simulink model "order2_math_model"  (R2021a)
settings: Solver=FixedStepAuto  StartTime=0.0  StopTime=15  FixedStep=1e-3  RelTol=1e-3
values from neighbouring files (symbols this model uses):
  K = [23.4125   -0.5709   44.4357   22.3907 -283.0923  379.2252]    [order2_all_observer_sfun.m]    (also in order2_calc.m = K2)
  K_lqr = lqr(A,B,Q,R)    [order2_calc.m]
settings Model: Creator=cc  LastModifiedBy=cc

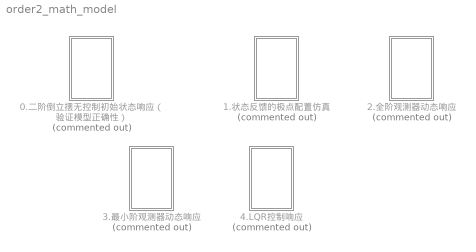
== system order2_math_model ==
  0.二阶倒立摆无控制初始状态响应（验证模型正确性） : Subsystem  Commented=on
  1.状态反馈的极点配置仿真 : Subsystem  Commented=on
  2.全阶观测器动态响应 : Subsystem  Commented=on
  3.最小阶观测器动态响应 : Subsystem  Commented=on
  4.LQR控制响应 : Subsystem  Commented=on

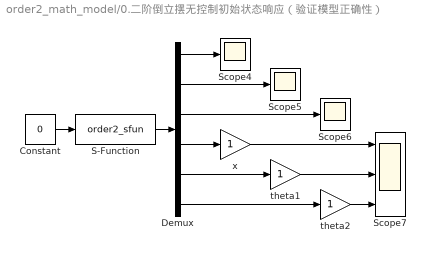
== system order2_math_model/0.二阶倒立摆无控制初始状态响应（验证模型正确性） ==
  Constant : Constant  Value=0
  Demux : Demux  Outputs=6
  S-Function : S-Function  FunctionName=order2_sfun  Parameters=0; 0; 0; 0; pi; 5/6*pi  SFunctionDeploymentMode=off  EnableBusSupport=off
  Scope4 : Scope
  Scope5 : Scope
  Scope6 : Scope
  Scope7 : Scope  NumInputPorts=3
  theta1 : Gain
  theta2 : Gain
  x : Gain
  wires:
  x/1 -> Scope7/1
  Demux/2 -> Scope5/1
  Constant/1 -> S-Function/1
  theta2/1 -> Scope7/3
  Demux/5 -> theta1/1
  theta1/1 -> Scope7/2
  Demux/6 -> theta2/1
  Demux/3 -> Scope6/1
  Demux/4 -> x/1
  S-Function/1 -> Demux/1
  Demux/1 -> Scope4/1

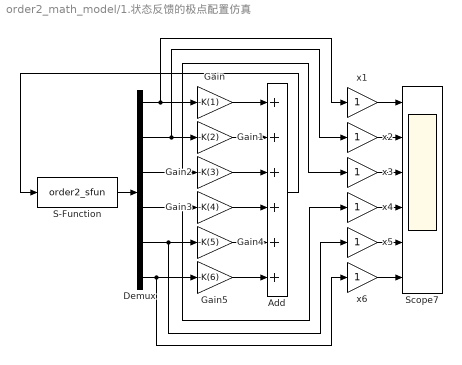
== system order2_math_model/1.状态反馈的极点配置仿真 ==
  Add : Sum  Inputs=++++++
  Demux : Demux  Outputs=6
  Gain : Gain  Gain=-K(1)
  Gain1 : Gain  Gain=-K(2)
  Gain2 : Gain  Gain=-K(3)
  Gain3 : Gain  Gain=-K(4)
  Gain4 : Gain  Gain=-K(5)
  Gain5 : Gain  Gain=-K(6)
  S-Function : S-Function  FunctionName=order2_sfun  Parameters=0; 0; 0; 0; 0; 5/180*pi  SFunctionDeploymentMode=off  EnableBusSupport=off
  Scope7 : Scope  NumInputPorts=6
  x{1..6} (6 alike) : Gain
  wires:
  S-Function/1 -> Demux/1
  Demux/1 -> x1/1, Gain/1
  Demux/2 -> Gain1/1, x2/1
  Demux/3 -> x3/1, Gain2/1
  Demux/4 -> x4/1, Gain3/1
  Demux/5 -> x5/1, Gain4/1
  Demux/6 -> x6/1, Gain5/1
  Gain/1 -> Add/1
  Gain1/1 -> Add/2
  Gain2/1 -> Add/3
  Gain3/1 -> Add/4
  Gain4/1 -> Add/5
  Gain5/1 -> Add/6
  Add/1 -> S-Function/1
  x1/1 -> Scope7/1
  x2/1 -> Scope7/2
  x3/1 -> Scope7/3
  x4/1 -> Scope7/4
  x5/1 -> Scope7/5
  x6/1 -> Scope7/6

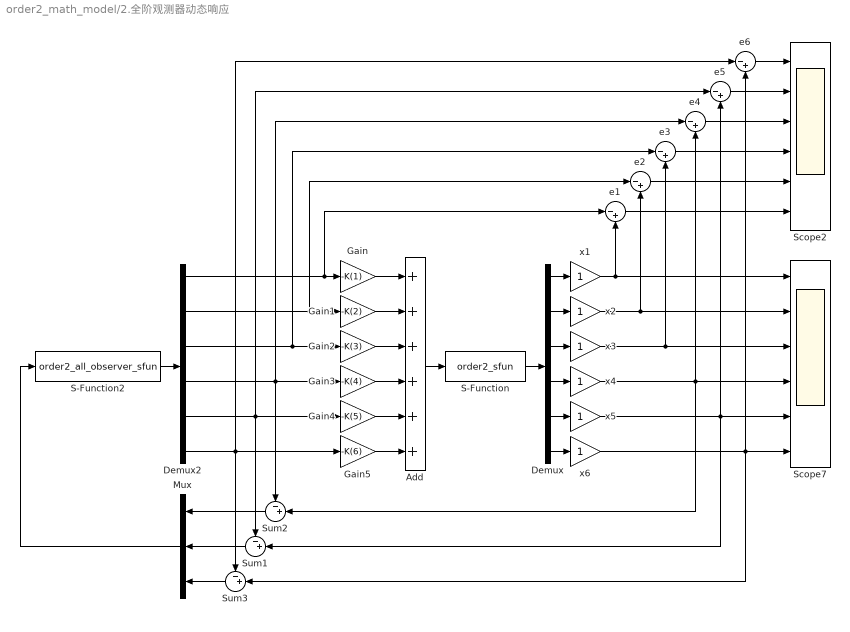
== system order2_math_model/2.全阶观测器动态响应 ==
  Add : Sum  Inputs=++++++
  Demux : Demux  Outputs=6
  Demux2 : Demux  Outputs=6
  Gain : Gain  Gain=-K(1)
  Gain1 : Gain  Gain=-K(2)
  Gain2 : Gain  Gain=-K(3)
  Gain3 : Gain  Gain=-K(4)
  Gain4 : Gain  Gain=-K(5)
  Gain5 : Gain  Gain=-K(6)
  Mux : Mux  Inputs=3
  S-Function : S-Function  FunctionName=order2_sfun  Parameters=0; 0; 0; 0; 0; 5/180*pi  SFunctionDeploymentMode=off  EnableBusSupport=off
  S-Function2 : S-Function  FunctionName=order2_all_observer_sfun  Parameters=0; 0; 0  SFunctionDeploymentMode=off  EnableBusSupport=off
  Scope2 : Scope  NumInputPorts=6
  Scope7 : Scope  NumInputPorts=6
  Sum1 : Sum  Inputs=-+|
  Sum2 : Sum  Inputs=-+|
  Sum3 : Sum  Inputs=-+|
  e{1..6} (6 alike) : Sum  Inputs=|-+
  x{1..6} (6 alike) : Gain
  wires:
  Demux/6 -> x6/1
  Gain/1 -> Add/1
  Gain1/1 -> Add/2
  Gain2/1 -> Add/3
  Gain3/1 -> Add/4
  Gain4/1 -> Add/5
  Gain5/1 -> Add/6
  Demux2/2 -> e2/1, Gain1/1
  Demux2/3 -> e3/1, Gain2/1
  Demux2/4 -> Gain3/1, e4/1, Sum2/1
  Demux2/5 -> Gain4/1, e5/1, Sum1/1
  Demux2/6 -> e6/1, Gain5/1, Sum3/1
  S-Function2/1 -> Demux2/1
  Demux2/1 -> e1/1, Gain/1
  Demux/4 -> x4/1
  Demux/5 -> x5/1
  Mux/1 -> S-Function2/1
  Demux/1 -> x1/1
  Demux/2 -> x2/1
  Demux/3 -> x3/1
  Sum2/1 -> Mux/1
  Sum1/1 -> Mux/2
  Sum3/1 -> Mux/3
  e3/1 -> Scope2/4
  e4/1 -> Scope2/3
  e5/1 -> Scope2/2
  e1/1 -> Scope2/6
  e2/1 -> Scope2/5
  e6/1 -> Scope2/1
  x1/1 -> Scope7/1, e1/2
  x3/1 -> Scope7/3, e3/2
  x4/1 -> Scope7/4, Sum2/2, e4/2
  x5/1 -> Scope7/5, Sum1/2, e5/2
  x6/1 -> Scope7/6, Sum3/2, e6/2
  x2/1 -> Scope7/2, e2/2
  Add/1 -> S-Function/1
  S-Function/1 -> Demux/1

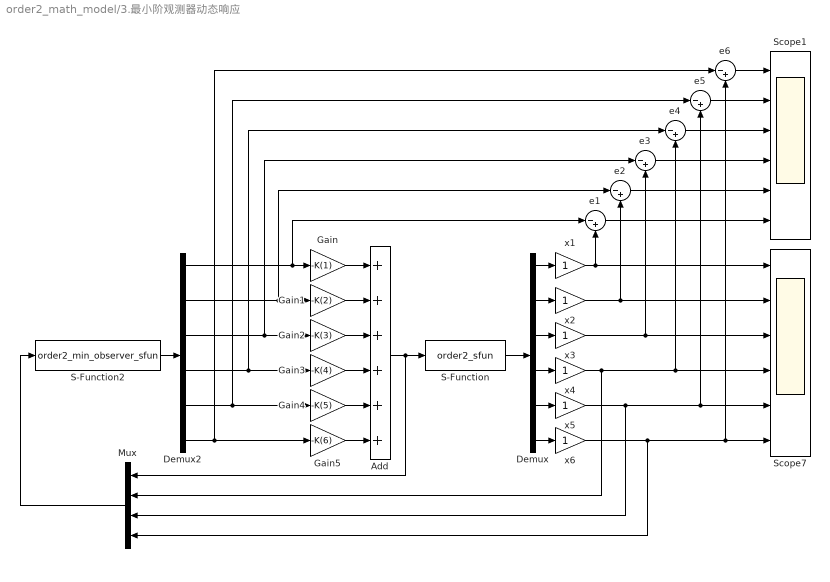
== system order2_math_model/3.最小阶观测器动态响应 ==
  Add : Sum  Inputs=++++++
  Demux : Demux  Outputs=6
  Demux2 : Demux  Outputs=6
  Gain : Gain  Gain=-K(1)
  Gain1 : Gain  Gain=-K(2)
  Gain2 : Gain  Gain=-K(3)
  Gain3 : Gain  Gain=-K(4)
  Gain4 : Gain  Gain=-K(5)
  Gain5 : Gain  Gain=-K(6)
  Mux : Mux
  S-Function : S-Function  FunctionName=order2_sfun  Parameters=0.05; 10/180*pi; 10/180*pi; 0; 0; 5/180*pi  SFunctionDeploymentMode=off  EnableBusSupport=off
  S-Function2 : S-Function  FunctionName=order2_min_observer_sfun  Parameters=0; 0; 5/180*pi; 0; 0; 0  SFunctionDeploymentMode=off  EnableBusSupport=off
  Scope1 : Scope  NumInputPorts=6
  Scope7 : Scope  NumInputPorts=6
  e{1..6} (6 alike) : Sum  Inputs=|-+
  x{1..6} (6 alike) : Gain
  wires:
  S-Function/1 -> Demux/1
  Demux/6 -> x6/1
  Gain/1 -> Add/1
  Gain1/1 -> Add/2
  Gain2/1 -> Add/3
  Gain3/1 -> Add/4
  Gain4/1 -> Add/5
  Gain5/1 -> Add/6
  Demux2/2 -> e2/1, Gain1/1
  Demux2/3 -> e3/1, Gain2/1
  Demux2/4 -> e4/1, Gain3/1
  Demux2/5 -> e5/1, Gain4/1
  Demux2/6 -> e6/1, Gain5/1
  S-Function2/1 -> Demux2/1
  Demux2/1 -> e1/1, Gain/1
  Demux/4 -> x4/1
  Demux/5 -> x5/1
  Add/1 -> S-Function/1, Mux/1
  Mux/1 -> S-Function2/1
  Demux/1 -> x1/1
  Demux/2 -> x2/1
  Demux/3 -> x3/1
  e1/1 -> Scope1/6
  e2/1 -> Scope1/5
  e3/1 -> Scope1/4
  e4/1 -> Scope1/3
  e5/1 -> Scope1/2
  x1/1 -> e1/2, Scope7/1
  x2/1 -> e2/2, Scope7/2
  x3/1 -> e3/2, Scope7/3
  x4/1 -> e4/2, Scope7/4, Mux/2
  x5/1 -> e5/2, Scope7/5, Mux/3
  x6/1 -> e6/2, Scope7/6, Mux/4
  e6/1 -> Scope1/1

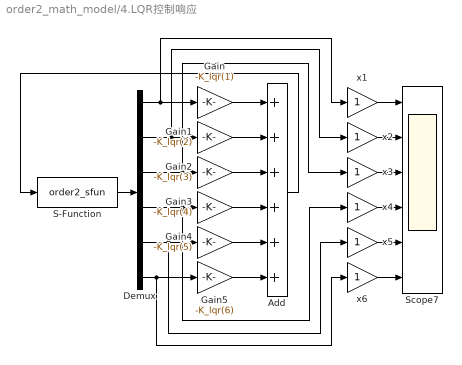
== system order2_math_model/4.LQR控制响应 ==
  Add : Sum  Inputs=++++++
  Demux : Demux  Outputs=6
  Gain : Gain  Gain=-K_lqr(1)
  Gain1 : Gain  Gain=-K_lqr(2)
  Gain2 : Gain  Gain=-K_lqr(3)
  Gain3 : Gain  Gain=-K_lqr(4)
  Gain4 : Gain  Gain=-K_lqr(5)
  Gain5 : Gain  Gain=-K_lqr(6)
  S-Function : S-Function  FunctionName=order2_sfun  Parameters=0; 0; 0; 0; 0; 5/180*pi  SFunctionDeploymentMode=off  EnableBusSupport=off
  Scope7 : Scope  NumInputPorts=6
  x{1..6} (6 alike) : Gain
  wires:
  S-Function/1 -> Demux/1
  Demux/1 -> x1/1, Gain/1
  Demux/2 -> Gain1/1, x2/1
  Demux/3 -> x3/1, Gain2/1
  Demux/4 -> x4/1, Gain3/1
  Demux/5 -> x5/1, Gain4/1
  Demux/6 -> x6/1, Gain5/1
  Gain/1 -> Add/1
  Gain1/1 -> Add/2
  Gain2/1 -> Add/3
  Gain3/1 -> Add/4
  Gain4/1 -> Add/5
  Gain5/1 -> Add/6
  Add/1 -> S-Function/1
  x1/1 -> Scope7/1
  x2/1 -> Scope7/2
  x3/1 -> Scope7/3
  x4/1 -> Scope7/4
  x5/1 -> Scope7/5
  x6/1 -> Scope7/6
